simulink model "CoolingTowerExample"  (Simulink 7.6)
settings: Solver=ode45  StartTime=0.0  StopTime=10*3600  RelTol=1e-3
libraries: carnot x3
settings Model: Creator=drhf  LastModifiedBy=drhf
settings CodeAppCC: CustomSymbolStrType=$N$R$M_T

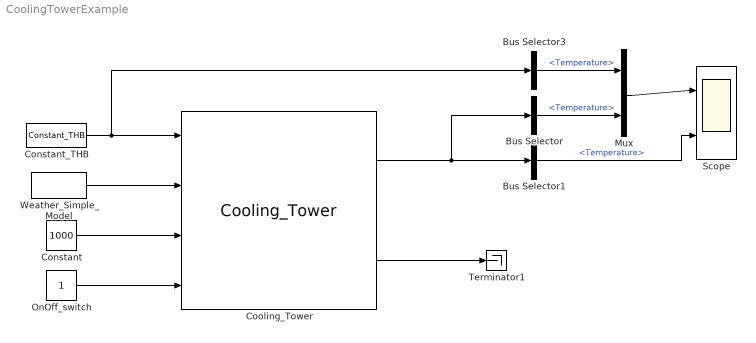
== system CoolingTowerExample ==
  Bus Selector : BusSelector  OutputSignals=Temperature
  Bus Selector1 : BusSelector  OutputSignals=Temperature
  Bus Selector3 : BusSelector  OutputSignals=Temperature
  Constant : Constant  Value=1000
  Constant_THB : carnot/Source/Simple/Constant_THB  SystemSampleTime=-1  t=15  mdot=1200/3600  p=1e5  mID=No Pressure Drop  fluid=water  mix=0  dia=0.02  hgt=0
  Cooling_Tower : carnot/Source/Chiller/Cooling_Tower  SystemSampleTime=-1
  Mux : Mux  Inputs=2
  OnOff_switch : Constant
      settings: OpenFcn=set_param(gcb,'value',num2str(1-str2num(get_param(gcb,'value'))))
  Scope : Scope  NumInputPorts=2
      settings: YMin=-5~-5  YMax=5~5
  Terminator1 : Terminator
  Weather_Simple_Model : carnot/Weather/Weather_Simple_Model  SystemSampleTime=-1  lat=60  Ibn=900  Idg=100  tamb=5  deltaTsky=-6  rh=50  precip="10e-3/24/3600           % 10 mm in 24 h"  cloud=0.125  p=1013e2  vw=1  wdir=270
  wires:
  Constant_THB/1 -> Bus Selector3/1, Cooling_Tower/1
  OnOff_switch/1 -> Cooling_Tower/4
  Bus Selector3/1 -> Mux/1  "<Temperature>"
  Mux/1 -> Scope/1
  Cooling_Tower/1 -> Bus Selector/1, Bus Selector1/1
  Bus Selector/1 -> Mux/2  "<Temperature>"
  Bus Selector1/1 -> Scope/2  "<Temperature>"
  Weather_Simple_Model/1 -> Cooling_Tower/2
  Constant/1 -> Cooling_Tower/3
  Cooling_Tower/2 -> Terminator1/1
